simulink model "acelerando_o_bloco_encoder"  (R2012b)
settings: Solver=ode3  StartTime=0.0  StopTime=10  FixedStep=1e-5  RelTol=1e-3
libraries: Encoder x1, simulink x1
settings Model: Creator=Juliano  LastModifiedBy=Juliano

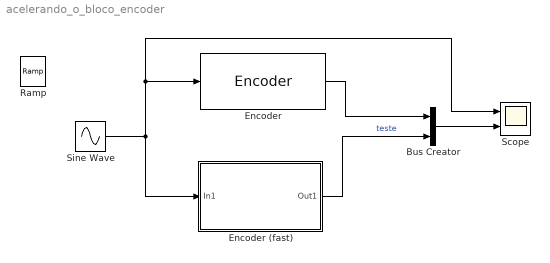
== system acelerando_o_bloco_encoder ==
  Bus Creator : BusCreator  Inputs=2
  Encoder : Encoder/Encoder  Nr=3000
  Encoder (fast) : Subsystem  mask{Nr=3000}
  Ramp : simulink/Sources/Ramp  slope=100  start=0  X0=0
  Scope : Scope  NumInputPorts=2
      settings: ShowLegends=on  YMin=-1000~-1000  YMax=1000~1100
  Sine Wave : Sin  Amplitude=01000  SampleTime=0
  wires:
  Encoder/1 -> Bus Creator/1
  Encoder (fast)/1(Out1) -> Bus Creator/2  "teste"
  Bus Creator/1 -> Scope/2
  Sine Wave/1 -> Encoder (fast)/1(In1), Scope/1, Encoder/1

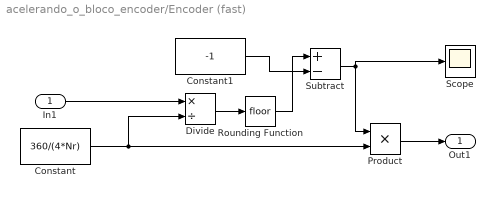
== system acelerando_o_bloco_encoder/Encoder (fast) ==
  In1 : Inport
  Constant : Constant  Value=360/(4*Nr)
  Constant1 : Constant  Value=-1
  Divide : Product  Inputs=*/
  Product : Product  RndMeth=Zero
  Rounding Function : Rounding
  Scope : Scope
  Subtract : Sum  Inputs=+-
  Out1 : Outport
  wires:
  Product/1 -> Out1/1
  Constant/1 -> Divide/2, Product/2
  In1/1 -> Divide/1
  Subtract/1 -> Product/1, Scope/1
  Divide/1 -> Rounding Function/1
  Rounding Function/1 -> Subtract/1
  Constant1/1 -> Subtract/2
